simulink model "CryoDetMultiChan_CMB"  (R2016b)
settings: Solver=ode45  StartTime=0.0  StopTime=400e-6  MaxStep=Tclk/4  RelTol=1e-3
values from neighbouring files (symbols this model uses):
  ds_axi = 16    [setupCryoFPGA_CMB.m]
  Fclk = Fadc    (= 307200000)    [setupCryoFPGA_CMB.m]
  lpf = tf(num,den)    [setupCryoFPGA_CMB.m]
  Tclk = 1/Fclk    (= 3.25520833333e-09)    [setupCryoFPGA_CMB.m]
  Ts = 1/Fs    (= 3.25520833333e-09)    [setupADCtoDACloopback.m]    (also in setupCryoFPGA_CMB.m)
undefined symbols (not defined in the file or in its folder): AXI4, i, Lite, xlipgetpartsetting
libraries: xbsIndex_r4 x2215, hdlsllib x6, simulink x3, CryoDetLib x2
(part 2 of 16)

== system CryoDetMultiChan_CMB/DspCore/DAC_fs_LO_Regs ==
  "dfs_LO 0 " : Inport
  dfs_LO 1 : Inport  Port=2
  dfs_LO 2 : Inport  Port=3
  dfs_LO 3 : Inport  Port=4
  dfs_LO 4 : Inport  Port=5
  dfs_LO 5 : Inport  Port=6
  dfs_LO 6 : Inport  Port=7
  dfs_LO 7 : Inport  Port=8
  dfs_LO 8 : Inport  Port=9
  dfs_LO 9 : Inport  Port=10
  dfs_LO 10 : Inport  Port=11
  dfs_LO 11 : Inport  Port=12
  dfs_LO 12 : Inport  Port=13
  dfs_LO 13 : Inport  Port=14
  dfs_LO 14 : Inport  Port=15
  dfs_LO 15 : Inport  Port=16
  BitBasher1 : xbsIndex_r4/BitBasher  bitexpr=a={b[15:0]}  display_expr=on  sr_1=a  arith_type1=Unsigned  bin_pt1=16  sr_2=2  arith_type2=Unsigned  bin_pt2=0  sr_3=3  arith_type3=Unsigned  bin_pt3=0  sr_4=4  arith_type4=Unsigned  bin_pt4=0  dbl_ovrd=off  block_type=bitbasher
  BitBasher{2..11,14,17..20} (15 alike) : xbsIndex_r4/BitBasher  bitexpr=a={b[24:0]}  display_expr=on  sr_1=a  arith_type1=Unsigned  bin_pt1=0  sr_2=2  arith_type2=Unsigned  bin_pt2=0  sr_3=3  arith_type3=Unsigned  bin_pt3=0  sr_4=4  arith_type4=Unsigned  bin_pt4=0  dbl_ovrd=off  block_type=bitbasher
  DSPcore_IO48 : xbsIndex_r4/Gateway In  gui_display_data_type=Fixed-point  arith_type=Unsigned  n_bits=32  bin_pt=0  preci_type=Single  exp_width=8  frac_width=24  rows=1  columns=1  quantization=Truncate  overflow=Wrap  period=Tclk*ds_axi  UseAsADC=off  ADCChannel='1'  interface=AXI4-Lite  automatic_assignment=off  address_offset=hex2dec('B00')  intf_name=''  intf_description=''  default_value=0  timing_constraint=None  locs_specified=off  LOCs={}  io_standard={}  inherit_from_input=off  hdl_port=on  dbl_ovrd=off  block_type=gatewayin
  DSPcore_IO49 : xbsIndex_r4/Gateway In  gui_display_data_type=Fixed-point  arith_type=Unsigned  n_bits=32  bin_pt=0  preci_type=Single  exp_width=8  frac_width=24  rows=1  columns=1  quantization=Truncate  overflow=Wrap  period=Tclk*ds_axi  UseAsADC=off  ADCChannel='1'  interface=AXI4-Lite  automatic_assignment=off  address_offset=hex2dec('B04')  intf_name=''  intf_description=''  default_value=0  timing_constraint=None  locs_specified=off  LOCs={}  io_standard={}  inherit_from_input=off  hdl_port=on  dbl_ovrd=off  block_type=gatewayin
  DSPcore_IO50 : xbsIndex_r4/Gateway In  gui_display_data_type=Fixed-point  arith_type=Unsigned  n_bits=32  bin_pt=0  preci_type=Single  exp_width=8  frac_width=24  rows=1  columns=1  quantization=Truncate  overflow=Wrap  period=Tclk*ds_axi  UseAsADC=off  ADCChannel='1'  interface=AXI4-Lite  automatic_assignment=off  address_offset=hex2dec('B28')  intf_name=''  intf_description=''  default_value=0  timing_constraint=None  locs_specified=off  LOCs={}  io_standard={}  inherit_from_input=off  hdl_port=on  dbl_ovrd=off  block_type=gatewayin
  DSPcore_IO51 : xbsIndex_r4/Gateway In  gui_display_data_type=Fixed-point  arith_type=Unsigned  n_bits=32  bin_pt=0  preci_type=Single  exp_width=8  frac_width=24  rows=1  columns=1  quantization=Truncate  overflow=Wrap  period=Tclk*ds_axi  UseAsADC=off  ADCChannel='1'  interface=AXI4-Lite  automatic_assignment=off  address_offset=hex2dec('B2C')  intf_name=''  intf_description=''  default_value=0  timing_constraint=None  locs_specified=off  LOCs={}  io_standard={}  inherit_from_input=off  hdl_port=on  dbl_ovrd=off  block_type=gatewayin
  DSPcore_IO52 : xbsIndex_r4/Gateway In  gui_display_data_type=Fixed-point  arith_type=Unsigned  n_bits=32  bin_pt=0  preci_type=Single  exp_width=8  frac_width=24  rows=1  columns=1  quantization=Truncate  overflow=Wrap  period=Tclk*ds_axi  UseAsADC=off  ADCChannel='1'  interface=AXI4-Lite  automatic_assignment=off  address_offset=hex2dec('B30')  intf_name=''  intf_description=''  default_value=0  timing_constraint=None  locs_specified=off  LOCs={}  io_standard={}  inherit_from_input=off  hdl_port=on  dbl_ovrd=off  block_type=gatewayin
  DSPcore_IO53 : xbsIndex_r4/Gateway In  gui_display_data_type=Fixed-point  arith_type=Unsigned  n_bits=32  bin_pt=0  preci_type=Single  exp_width=8  frac_width=24  rows=1  columns=1  quantization=Truncate  overflow=Wrap  period=Tclk*ds_axi  UseAsADC=off  ADCChannel='1'  interface=AXI4-Lite  automatic_assignment=off  address_offset=hex2dec('B34')  intf_name=''  intf_description=''  default_value=0  timing_constraint=None  locs_specified=off  LOCs={}  io_standard={}  inherit_from_input=off  hdl_port=on  dbl_ovrd=off  block_type=gatewayin
  DSPcore_IO54 : xbsIndex_r4/Gateway In  gui_display_data_type=Fixed-point  arith_type=Unsigned  n_bits=32  bin_pt=0  preci_type=Single  exp_width=8  frac_width=24  rows=1  columns=1  quantization=Truncate  overflow=Wrap  period=Tclk*ds_axi  UseAsADC=off  ADCChannel='1'  interface=AXI4-Lite  automatic_assignment=off  address_offset=hex2dec('B38')  intf_name=''  intf_description=''  default_value=0  timing_constraint=None  locs_specified=off  LOCs={}  io_standard={}  inherit_from_input=off  hdl_port=on  dbl_ovrd=off  block_type=gatewayin
  DSPcore_IO55 : xbsIndex_r4/Gateway In  gui_display_data_type=Fixed-point  arith_type=Unsigned  n_bits=32  bin_pt=0  preci_type=Single  exp_width=8  frac_width=24  rows=1  columns=1  quantization=Truncate  overflow=Wrap  period=Tclk*ds_axi  UseAsADC=off  ADCChannel='1'  interface=AXI4-Lite  automatic_assignment=off  address_offset=hex2dec('B3C')  intf_name=''  intf_description=''  default_value=0  timing_constraint=None  locs_specified=off  LOCs={}  io_standard={}  inherit_from_input=off  hdl_port=on  dbl_ovrd=off  block_type=gatewayin
  DSPcore_IO56 : xbsIndex_r4/Gateway In  gui_display_data_type=Fixed-point  arith_type=Unsigned  n_bits=32  bin_pt=0  preci_type=Single  exp_width=8  frac_width=24  rows=1  columns=1  quantization=Truncate  overflow=Wrap  period=Tclk*ds_axi  UseAsADC=off  ADCChannel='1'  interface=AXI4-Lite  automatic_assignment=off  address_offset=hex2dec('B08')  intf_name=''  intf_description=''  default_value=0  timing_constraint=None  locs_specified=off  LOCs={}  io_standard={}  inherit_from_input=off  hdl_port=on  dbl_ovrd=off  block_type=gatewayin
  DSPcore_IO57 : xbsIndex_r4/Gateway In  gui_display_data_type=Fixed-point  arith_type=Unsigned  n_bits=32  bin_pt=0  preci_type=Single  exp_width=8  frac_width=24  rows=1  columns=1  quantization=Truncate  overflow=Wrap  period=Tclk*ds_axi  UseAsADC=off  ADCChannel='1'  interface=AXI4-Lite  automatic_assignment=off  address_offset=hex2dec('B0C')  intf_name=''  intf_description=''  default_value=0  timing_constraint=None  locs_specified=off  LOCs={}  io_standard={}  inherit_from_input=off  hdl_port=on  dbl_ovrd=off  block_type=gatewayin
  DSPcore_IO58 : xbsIndex_r4/Gateway In  gui_display_data_type=Fixed-point  arith_type=Unsigned  n_bits=32  bin_pt=0  preci_type=Single  exp_width=8  frac_width=24  rows=1  columns=1  quantization=Truncate  overflow=Wrap  period=Tclk*ds_axi  UseAsADC=off  ADCChannel='1'  interface=AXI4-Lite  automatic_assignment=off  address_offset=hex2dec('B10')  intf_name=''  intf_description=''  default_value=0  timing_constraint=None  locs_specified=off  LOCs={}  io_standard={}  inherit_from_input=off  hdl_port=on  dbl_ovrd=off  block_type=gatewayin
  DSPcore_IO59 : xbsIndex_r4/Gateway In  gui_display_data_type=Fixed-point  arith_type=Unsigned  n_bits=32  bin_pt=0  preci_type=Single  exp_width=8  frac_width=24  rows=1  columns=1  quantization=Truncate  overflow=Wrap  period=Tclk*ds_axi  UseAsADC=off  ADCChannel='1'  interface=AXI4-Lite  automatic_assignment=off  address_offset=hex2dec('B14')  intf_name=''  intf_description=''  default_value=0  timing_constraint=None  locs_specified=off  LOCs={}  io_standard={}  inherit_from_input=off  hdl_port=on  dbl_ovrd=off  block_type=gatewayin
  DSPcore_IO60 : xbsIndex_r4/Gateway In  gui_display_data_type=Fixed-point  arith_type=Unsigned  n_bits=32  bin_pt=0  preci_type=Single  exp_width=8  frac_width=24  rows=1  columns=1  quantization=Truncate  overflow=Wrap  period=Tclk*ds_axi  UseAsADC=off  ADCChannel='1'  interface=AXI4-Lite  automatic_assignment=off  address_offset=hex2dec('B18')  intf_name=''  intf_description=''  default_value=0  timing_constraint=None  locs_specified=off  LOCs={}  io_standard={}  inherit_from_input=off  hdl_port=on  dbl_ovrd=off  block_type=gatewayin
  DSPcore_IO61 : xbsIndex_r4/Gateway In  gui_display_data_type=Fixed-point  arith_type=Unsigned  n_bits=32  bin_pt=0  preci_type=Single  exp_width=8  frac_width=24  rows=1  columns=1  quantization=Truncate  overflow=Wrap  period=Tclk*ds_axi  UseAsADC=off  ADCChannel='1'  interface=AXI4-Lite  automatic_assignment=off  address_offset=hex2dec('B1C')  intf_name=''  intf_description=''  default_value=0  timing_constraint=None  locs_specified=off  LOCs={}  io_standard={}  inherit_from_input=off  hdl_port=on  dbl_ovrd=off  block_type=gatewayin
  DSPcore_IO62 : xbsIndex_r4/Gateway In  gui_display_data_type=Fixed-point  arith_type=Unsigned  n_bits=32  bin_pt=0  preci_type=Single  exp_width=8  frac_width=24  rows=1  columns=1  quantization=Truncate  overflow=Wrap  period=Tclk*ds_axi  UseAsADC=off  ADCChannel='1'  interface=AXI4-Lite  automatic_assignment=off  address_offset=hex2dec('B20')  intf_name=''  intf_description=''  default_value=0  timing_constraint=None  locs_specified=off  LOCs={}  io_standard={}  inherit_from_input=off  hdl_port=on  dbl_ovrd=off  block_type=gatewayin
  DSPcore_IO63 : xbsIndex_r4/Gateway In  gui_display_data_type=Fixed-point  arith_type=Unsigned  n_bits=32  bin_pt=0  preci_type=Single  exp_width=8  frac_width=24  rows=1  columns=1  quantization=Truncate  overflow=Wrap  period=Tclk*ds_axi  UseAsADC=off  ADCChannel='1'  interface=AXI4-Lite  automatic_assignment=off  address_offset=hex2dec('B24')  intf_name=''  intf_description=''  default_value=0  timing_constraint=None  locs_specified=off  LOCs={}  io_standard={}  inherit_from_input=off  hdl_port=on  dbl_ovrd=off  block_type=gatewayin
  F{0..3} (4 alike) : Display
  Gateway Out{,2..4} (4 alike) : xbsIndex_r4/Gateway Out  inherit_from_input=on  hdl_port=off  rows=1  columns=1  UseAsDAC=off  DACChannel='1'  interface=None  automatic_assignment=on  address_offset=hex2dec('00')  intf_name=''  intf_description=''  timing_constraint=None  locs_specified=off  LOCs={}  io_standard={}  block_type=gatewayout
  pipeline_2r : Subsystem
  pipeline_2r1 : Subsystem
  pipeline_2r10 : Subsystem
  pipeline_2r11 : Subsystem
  pipeline_2r12 : Subsystem
  pipeline_2r13 : Subsystem
  pipeline_2r14 : Subsystem
  pipeline_2r15 : Subsystem
  pipeline_2r2 : Subsystem
  pipeline_2r3 : Subsystem
  pipeline_2r4 : Subsystem
  pipeline_2r5 : Subsystem
  pipeline_2r6 : Subsystem
  pipeline_2r7 : Subsystem
  pipeline_2r8 : Subsystem
  pipeline_2r9 : Subsystem
  tag scope: dfs_LO0=global, dfs_LO10=global, dfs_LO11=global, dfs_LO12=global, dfs_LO13=global, dfs_LO14=global, dfs_LO15=global, dfs_LO1=global, dfs_LO2=global, dfs_LO3=global, dfs_LO4=global, dfs_LO5=global, dfs_LO6=global, dfs_LO7=global, dfs_LO8=global, dfs_LO9=global
  wires:
  dfs_LO 14/1 -> DSPcore_IO54/1
  BitBasher5/1 -> [dfs_LO4]
  DSPcore_IO58/1 -> pipeline_2r4/1(In1)
  BitBasher17/1 -> [dfs_LO13]
  dfs_LO 13/1 -> DSPcore_IO53/1
  DSPcore_IO59/1 -> pipeline_2r5/1(In1)
  dfs_LO 15/1 -> DSPcore_IO55/1
  BitBasher11/1 -> [dfs_LO10]
  dfs_LO 7/1 -> DSPcore_IO61/1
  dfs_LO 11/1 -> DSPcore_IO51/1
  dfs_LO 9/1 -> DSPcore_IO63/1
  Gateway Out4/1 -> F3/1
  BitBasher4/1 -> [dfs_LO3], Gateway Out4/1
  dfs_LO 5/1 -> DSPcore_IO59/1
  DSPcore_IO55/1 -> pipeline_2r15/1(In1)
  DSPcore_IO53/1 -> pipeline_2r13/1(In1)
  DSPcore_IO63/1 -> pipeline_2r9/1(In1)
  BitBasher6/1 -> [dfs_LO5]
  dfs_LO 8/1 -> DSPcore_IO62/1
  DSPcore_IO52/1 -> pipeline_2r12/1(In1)
  BitBasher20/1 -> [dfs_LO12]
  DSPcore_IO57/1 -> pipeline_2r3/1(In1)
  dfs_LO 4/1 -> DSPcore_IO58/1
  Gateway Out2/1 -> F1/1
  BitBasher2/1 -> [dfs_LO1], Gateway Out2/1
  DSPcore_IO62/1 -> pipeline_2r8/1(In1)
  BitBasher14/1 -> [dfs_LO11]
  BitBasher19/1 -> [dfs_LO15]
  dfs_LO 10/1 -> DSPcore_IO50/1
  BitBasher10/1 -> [dfs_LO9]
  DSPcore_IO51/1 -> pipeline_2r11/1(In1)
  DSPcore_IO56/1 -> pipeline_2r2/1(In1)
  dfs_LO 2/1 -> DSPcore_IO56/1
  Gateway Out3/1 -> F2/1
  BitBasher3/1 -> [dfs_LO2], Gateway Out3/1
  DSPcore_IO54/1 -> pipeline_2r14/1(In1)
  DSPcore_IO49/1 -> pipeline_2r1/1(In1)
  dfs_LO 1/1 -> DSPcore_IO49/1
  BitBasher9/1 -> [dfs_LO8]
  DSPcore_IO61/1 -> pipeline_2r7/1(In1)
  BitBasher18/1 -> [dfs_LO14]
  DSPcore_IO50/1 -> pipeline_2r10/1(In1)
  dfs_LO 6/1 -> DSPcore_IO60/1
  dfs_LO 3/1 -> DSPcore_IO57/1
  "dfs_LO 0 "/1 -> DSPcore_IO48/1
  Gateway Out/1 -> F0/1
  BitBasher1/1 -> [dfs_LO0], Gateway Out/1
  DSPcore_IO48/1 -> pipeline_2r/1(In1)
  BitBasher7/1 -> [dfs_LO6]
  BitBasher8/1 -> [dfs_LO7]
  dfs_LO 12/1 -> DSPcore_IO52/1
  DSPcore_IO60/1 -> pipeline_2r6/1(In1)
  pipeline_2r/1(Out1) -> BitBasher1/1
  pipeline_2r1/1(Out1) -> BitBasher2/1
  pipeline_2r2/1(Out1) -> BitBasher3/1
  pipeline_2r3/1(Out1) -> BitBasher4/1
  pipeline_2r5/1(Out1) -> BitBasher6/1
  pipeline_2r4/1(Out1) -> BitBasher5/1
  pipeline_2r6/1(Out1) -> BitBasher7/1
  pipeline_2r7/1(Out1) -> BitBasher8/1
  pipeline_2r9/1(Out1) -> BitBasher10/1
  pipeline_2r10/1(Out1) -> BitBasher11/1
  pipeline_2r8/1(Out1) -> BitBasher9/1
  pipeline_2r11/1(Out1) -> BitBasher14/1
  pipeline_2r13/1(Out1) -> BitBasher17/1
  pipeline_2r14/1(Out1) -> BitBasher18/1
  pipeline_2r12/1(Out1) -> BitBasher20/1
  pipeline_2r15/1(Out1) -> BitBasher19/1

== system CryoDetMultiChan_CMB/DspCore/FTA_Ch0 ==
  note: Band B is not used for now..
  note: reference
  ADCin_A : Inport
  ADCin_B : Inport  Port=2
  ADC_IQ_Swap : Subsystem
  DAC_Output_Fmt : Subsystem
  Goto Tag Visibility : GotoTagVisibility  GotoTag=freqBus
  Goto Tag Visibility1 : GotoTagVisibility  GotoTag=dphiBus
  Goto Tag Visibility2 : GotoTagVisibility  GotoTag=dFbus
  RF switch : Subsystem
  Ref Delay : Subsystem
  SixteenLineUDC 0 : Subsystem
  Terminator : Terminator
  Terminator1 : Terminator
  dF : Subsystem
  dphi : Subsystem
  loopFilter : Subsystem
  shiftFreq : Subsystem
  twelveLineUDC 1 : Subsystem
  DAC_I_out : Outport
  DAC_Q_out : Outport  Port=2
  wires:
  twelveLineUDC 1/1(Out1) -> Terminator/1
  SixteenLineUDC 0/1(toDAC) -> RF switch/1(In1)
  SixteenLineUDC 0/2(demodulated) -> dF/1(In1)
  dF/1(Out1) -> loopFilter/1(In1)
  loopFilter/1(Out1) -> dphi/1(In1)
  ADCin_B/1 -> Terminator1/1
  [Band1_IQ_In_Swap] -> ADC_IQ_Swap/1(Swap_en)
  ADCin_A/1 -> ADC_IQ_Swap/2(ADC_in)
  ADC_IQ_Swap/1(ADC_I_out) -> SixteenLineUDC 0/1(ADC_I_in)
  ADC_IQ_Swap/2(ADC_Q_out) -> SixteenLineUDC 0/2(ADC_Q_in)
  shiftFreq/1(Out1) -> DAC_Output_Fmt/1(In1)
  DAC_Output_Fmt/1(Out_Q) -> DAC_Q_out/1
  DAC_Output_Fmt/2(Out_I) -> DAC_I_out/1
  Ref Delay/1(Out_Q) -> SixteenLineUDC 0/4(REF_Q_in1)
  Ref Delay/2(Out_I) -> SixteenLineUDC 0/3(REF_I_in1)
  RF switch/1(to_DAC) -> shiftFreq/1(In1)
  RF switch/2(to_REF) -> Ref Delay/1(In1)

== system CryoDetMultiChan_CMB/DspCore/FTA_Ch1 ==
  note: FTA Ch1
      | Only a pass thu for now...
      |
      | Note that this type of 1:1 connection ONLY works
      | when the ADC is in Single-Band Complex mode b/c
      | of how the adc data is mapped.
      | This is here for testing only.
  ADCin_A : Inport
  ADCin_B : Inport  Port=2
  DAC_I_out : Outport
  DAC_Q_out : Outport  Port=2
  wires:
  ADCin_A/1 -> DAC_I_out/1
  ADCin_B/1 -> DAC_Q_out/1

== system CryoDetMultiChan_CMB/DspCore/Initial_Freq_Regs ==
  "Fi 0 " : Inport
  Fi 1 : Inport  Port=2
  Fi 2 : Inport  Port=3
  Fi 3 : Inport  Port=4
  Fi 4 : Inport  Port=5
  Fi 5 : Inport  Port=6
  Fi 6 : Inport  Port=7
  Fi 7 : Inport  Port=8
  Fi 8 : Inport  Port=9
  Fi 9 : Inport  Port=10
  Fi 10 : Inport  Port=11
  Fi 11 : Inport  Port=12
  Fi 12 : Inport  Port=13
  Fi 13 : Inport  Port=14
  Fi 14 : Inport  Port=15
  Fi 15 : Inport  Port=16
  BitBasher{1..11,14,17..20} (16 alike) : xbsIndex_r4/BitBasher  bitexpr=a={b[24:0]}  display_expr=on  sr_1=a  arith_type1=Unsigned  bin_pt1=0  sr_2=2  arith_type2=Unsigned  bin_pt2=0  sr_3=3  arith_type3=Unsigned  bin_pt3=0  sr_4=4  arith_type4=Unsigned  bin_pt4=0  dbl_ovrd=off  block_type=bitbasher
  DSPcore_IO : xbsIndex_r4/Gateway In  gui_display_data_type=Fixed-point  arith_type=Unsigned  n_bits=32  bin_pt=0  preci_type=Single  exp_width=8  frac_width=24  rows=1  columns=1  quantization=Truncate  overflow=Wrap  period=Tclk*ds_axi  UseAsADC=off  ADCChannel='1'  interface=AXI4-Lite  automatic_assignment=off  address_offset=hex2dec('900')  intf_name=''  intf_description=''  default_value=0  timing_constraint=None  locs_specified=off  LOCs={}  io_standard={}  inherit_from_input=off  hdl_port=on  dbl_ovrd=off  block_type=gatewayin
  DSPcore_IO1 : xbsIndex_r4/Gateway In  gui_display_data_type=Fixed-point  arith_type=Unsigned  n_bits=32  bin_pt=0  preci_type=Single  exp_width=8  frac_width=24  rows=1  columns=1  quantization=Truncate  overflow=Wrap  period=Tclk*ds_axi  UseAsADC=off  ADCChannel='1'  interface=AXI4-Lite  automatic_assignment=off  address_offset=hex2dec('904')  intf_name=''  intf_description=''  default_value=0  timing_constraint=None  locs_specified=off  LOCs={}  io_standard={}  inherit_from_input=off  hdl_port=on  dbl_ovrd=off  block_type=gatewayin
  DSPcore_IO10 : xbsIndex_r4/Gateway In  gui_display_data_type=Fixed-point  arith_type=Unsigned  n_bits=32  bin_pt=0  preci_type=Single  exp_width=8  frac_width=24  rows=1  columns=1  quantization=Truncate  overflow=Wrap  period=Tclk*ds_axi  UseAsADC=off  ADCChannel='1'  interface=AXI4-Lite  automatic_assignment=off  address_offset=hex2dec('928')  intf_name=''  intf_description=''  default_value=0  timing_constraint=None  locs_specified=off  LOCs={}  io_standard={}  inherit_from_input=off  hdl_port=on  dbl_ovrd=off  block_type=gatewayin
  DSPcore_IO11 : xbsIndex_r4/Gateway In  gui_display_data_type=Fixed-point  arith_type=Unsigned  n_bits=32  bin_pt=0  preci_type=Single  exp_width=8  frac_width=24  rows=1  columns=1  quantization=Truncate  overflow=Wrap  period=Tclk*ds_axi  UseAsADC=off  ADCChannel='1'  interface=AXI4-Lite  automatic_assignment=off  address_offset=hex2dec('92C')  intf_name=''  intf_description=''  default_value=0  timing_constraint=None  locs_specified=off  LOCs={}  io_standard={}  inherit_from_input=off  hdl_port=on  dbl_ovrd=off  block_type=gatewayin
  DSPcore_IO12 : xbsIndex_r4/Gateway In  gui_display_data_type=Fixed-point  arith_type=Unsigned  n_bits=32  bin_pt=0  preci_type=Single  exp_width=8  frac_width=24  rows=1  columns=1  quantization=Truncate  overflow=Wrap  period=Tclk*ds_axi  UseAsADC=off  ADCChannel='1'  interface=AXI4-Lite  automatic_assignment=off  address_offset=hex2dec('930')  intf_name=''  intf_description=''  default_value=0  timing_constraint=None  locs_specified=off  LOCs={}  io_standard={}  inherit_from_input=off  hdl_port=on  dbl_ovrd=off  block_type=gatewayin
  DSPcore_IO13 : xbsIndex_r4/Gateway In  gui_display_data_type=Fixed-point  arith_type=Unsigned  n_bits=32  bin_pt=0  preci_type=Single  exp_width=8  frac_width=24  rows=1  columns=1  quantization=Truncate  overflow=Wrap  period=Tclk*ds_axi  UseAsADC=off  ADCChannel='1'  interface=AXI4-Lite  automatic_assignment=off  address_offset=hex2dec('934')  intf_name=''  intf_description=''  default_value=0  timing_constraint=None  locs_specified=off  LOCs={}  io_standard={}  inherit_from_input=off  hdl_port=on  dbl_ovrd=off  block_type=gatewayin
  DSPcore_IO14 : xbsIndex_r4/Gateway In  gui_display_data_type=Fixed-point  arith_type=Unsigned  n_bits=32  bin_pt=0  preci_type=Single  exp_width=8  frac_width=24  rows=1  columns=1  quantization=Truncate  overflow=Wrap  period=Tclk*ds_axi  UseAsADC=off  ADCChannel='1'  interface=AXI4-Lite  automatic_assignment=off  address_offset=hex2dec('938')  intf_name=''  intf_description=''  default_value=0  timing_constraint=None  locs_specified=off  LOCs={}  io_standard={}  inherit_from_input=off  hdl_port=on  dbl_ovrd=off  block_type=gatewayin
  DSPcore_IO15 : xbsIndex_r4/Gateway In  gui_display_data_type=Fixed-point  arith_type=Unsigned  n_bits=32  bin_pt=0  preci_type=Single  exp_width=8  frac_width=24  rows=1  columns=1  quantization=Truncate  overflow=Wrap  period=Tclk*ds_axi  UseAsADC=off  ADCChannel='1'  interface=AXI4-Lite  automatic_assignment=off  address_offset=hex2dec('93C')  intf_name=''  intf_description=''  default_value=0  timing_constraint=None  locs_specified=off  LOCs={}  io_standard={}  inherit_from_input=off  hdl_port=on  dbl_ovrd=off  block_type=gatewayin
  DSPcore_IO2 : xbsIndex_r4/Gateway In  gui_display_data_type=Fixed-point  arith_type=Unsigned  n_bits=32  bin_pt=0  preci_type=Single  exp_width=8  frac_width=24  rows=1  columns=1  quantization=Truncate  overflow=Wrap  period=Tclk*ds_axi  UseAsADC=off  ADCChannel='1'  interface=AXI4-Lite  automatic_assignment=off  address_offset=hex2dec('908')  intf_name=''  intf_description=''  default_value=0  timing_constraint=None  locs_specified=off  LOCs={}  io_standard={}  inherit_from_input=off  hdl_port=on  dbl_ovrd=off  block_type=gatewayin
  DSPcore_IO3 : xbsIndex_r4/Gateway In  gui_display_data_type=Fixed-point  arith_type=Unsigned  n_bits=32  bin_pt=0  preci_type=Single  exp_width=8  frac_width=24  rows=1  columns=1  quantization=Truncate  overflow=Wrap  period=Tclk*ds_axi  UseAsADC=off  ADCChannel='1'  interface=AXI4-Lite  automatic_assignment=off  address_offset=hex2dec('90C')  intf_name=''  intf_description=''  default_value=0  timing_constraint=None  locs_specified=off  LOCs={}  io_standard={}  inherit_from_input=off  hdl_port=on  dbl_ovrd=off  block_type=gatewayin
  DSPcore_IO4 : xbsIndex_r4/Gateway In  gui_display_data_type=Fixed-point  arith_type=Unsigned  n_bits=32  bin_pt=0  preci_type=Single  exp_width=8  frac_width=24  rows=1  columns=1  quantization=Truncate  overflow=Wrap  period=Tclk*ds_axi  UseAsADC=off  ADCChannel='1'  interface=AXI4-Lite  automatic_assignment=off  address_offset=hex2dec('910')  intf_name=''  intf_description=''  default_value=0  timing_constraint=None  locs_specified=off  LOCs={}  io_standard={}  inherit_from_input=off  hdl_port=on  dbl_ovrd=off  block_type=gatewayin
  DSPcore_IO5 : xbsIndex_r4/Gateway In  gui_display_data_type=Fixed-point  arith_type=Unsigned  n_bits=32  bin_pt=0  preci_type=Single  exp_width=8  frac_width=24  rows=1  columns=1  quantization=Truncate  overflow=Wrap  period=Tclk*ds_axi  UseAsADC=off  ADCChannel='1'  interface=AXI4-Lite  automatic_assignment=off  address_offset=hex2dec('914')  intf_name=''  intf_description=''  default_value=0  timing_constraint=None  locs_specified=off  LOCs={}  io_standard={}  inherit_from_input=off  hdl_port=on  dbl_ovrd=off  block_type=gatewayin
  DSPcore_IO6 : xbsIndex_r4/Gateway In  gui_display_data_type=Fixed-point  arith_type=Unsigned  n_bits=32  bin_pt=0  preci_type=Single  exp_width=8  frac_width=24  rows=1  columns=1  quantization=Truncate  overflow=Wrap  period=Tclk*ds_axi  UseAsADC=off  ADCChannel='1'  interface=AXI4-Lite  automatic_assignment=off  address_offset=hex2dec('918')  intf_name=''  intf_description=''  default_value=0  timing_constraint=None  locs_specified=off  LOCs={}  io_standard={}  inherit_from_input=off  hdl_port=on  dbl_ovrd=off  block_type=gatewayin
  DSPcore_IO7 : xbsIndex_r4/Gateway In  gui_display_data_type=Fixed-point  arith_type=Unsigned  n_bits=32  bin_pt=0  preci_type=Single  exp_width=8  frac_width=24  rows=1  columns=1  quantization=Truncate  overflow=Wrap  period=Tclk*ds_axi  UseAsADC=off  ADCChannel='1'  interface=AXI4-Lite  automatic_assignment=off  address_offset=hex2dec('91C')  intf_name=''  intf_description=''  default_value=0  timing_constraint=None  locs_specified=off  LOCs={}  io_standard={}  inherit_from_input=off  hdl_port=on  dbl_ovrd=off  block_type=gatewayin
  DSPcore_IO8 : xbsIndex_r4/Gateway In  gui_display_data_type=Fixed-point  arith_type=Unsigned  n_bits=32  bin_pt=0  preci_type=Single  exp_width=8  frac_width=24  rows=1  columns=1  quantization=Truncate  overflow=Wrap  period=Tclk*ds_axi  UseAsADC=off  ADCChannel='1'  interface=AXI4-Lite  automatic_assignment=off  address_offset=hex2dec('920')  intf_name=''  intf_description=''  default_value=0  timing_constraint=None  locs_specified=off  LOCs={}  io_standard={}  inherit_from_input=off  hdl_port=on  dbl_ovrd=off  block_type=gatewayin
  DSPcore_IO9 : xbsIndex_r4/Gateway In  gui_display_data_type=Fixed-point  arith_type=Unsigned  n_bits=32  bin_pt=0  preci_type=Single  exp_width=8  frac_width=24  rows=1  columns=1  quantization=Truncate  overflow=Wrap  period=Tclk*ds_axi  UseAsADC=off  ADCChannel='1'  interface=AXI4-Lite  automatic_assignment=off  address_offset=hex2dec('924')  intf_name=''  intf_description=''  default_value=0  timing_constraint=None  locs_specified=off  LOCs={}  io_standard={}  inherit_from_input=off  hdl_port=on  dbl_ovrd=off  block_type=gatewayin
  F{0..3} (4 alike) : Display
  Gateway Out{,2..4} (4 alike) : xbsIndex_r4/Gateway Out  inherit_from_input=on  hdl_port=off  rows=1  columns=1  UseAsDAC=off  DACChannel='1'  interface=None  automatic_assignment=on  address_offset=hex2dec('00')  intf_name=''  intf_description=''  timing_constraint=None  locs_specified=off  LOCs={}  io_standard={}  block_type=gatewayout
  pipeline_2r : Subsystem
  pipeline_2r1 : Subsystem
  pipeline_2r10 : Subsystem
  pipeline_2r11 : Subsystem
  pipeline_2r12 : Subsystem
  pipeline_2r13 : Subsystem
  pipeline_2r14 : Subsystem
  pipeline_2r15 : Subsystem
  pipeline_2r2 : Subsystem
  pipeline_2r3 : Subsystem
  pipeline_2r4 : Subsystem
  pipeline_2r5 : Subsystem
  pipeline_2r6 : Subsystem
  pipeline_2r7 : Subsystem
  pipeline_2r8 : Subsystem
  pipeline_2r9 : Subsystem
  tag scope: F0=global, F10=global, F11=global, F12=global, F13=global, F14=global, F15=global, F1=global, F2=global, F3=global, F4=global, F5=global, F6=global, F7=global, F8=global, F9=global
  wires:
  Fi 14/1 -> DSPcore_IO14/1
  BitBasher5/1 -> [F4]
  DSPcore_IO4/1 -> pipeline_2r4/1(In1)
  BitBasher17/1 -> [F13]
  Fi 13/1 -> DSPcore_IO13/1
  DSPcore_IO5/1 -> pipeline_2r5/1(In1)
  Fi 15/1 -> DSPcore_IO15/1
  BitBasher11/1 -> [F10]
  Fi 7/1 -> DSPcore_IO7/1
  Fi 11/1 -> DSPcore_IO11/1
  Fi 9/1 -> DSPcore_IO9/1
  Gateway Out4/1 -> F3/1
  BitBasher4/1 -> Gateway Out4/1, [F3]
  Fi 5/1 -> DSPcore_IO5/1
  DSPcore_IO15/1 -> pipeline_2r15/1(In1)
  DSPcore_IO13/1 -> pipeline_2r13/1(In1)
  DSPcore_IO9/1 -> pipeline_2r9/1(In1)
  BitBasher6/1 -> [F5]
  Fi 8/1 -> DSPcore_IO8/1
  DSPcore_IO12/1 -> pipeline_2r12/1(In1)
  BitBasher20/1 -> [F12]
  DSPcore_IO3/1 -> pipeline_2r3/1(In1)
  Fi 4/1 -> DSPcore_IO4/1
  Gateway Out2/1 -> F1/1
  BitBasher2/1 -> [F1], Gateway Out2/1
  DSPcore_IO8/1 -> pipeline_2r8/1(In1)
  BitBasher14/1 -> [F11]
  BitBasher19/1 -> [F15]
  Fi 10/1 -> DSPcore_IO10/1
  BitBasher10/1 -> [F9]
  DSPcore_IO11/1 -> pipeline_2r11/1(In1)
  DSPcore_IO2/1 -> pipeline_2r2/1(In1)
  Fi 2/1 -> DSPcore_IO2/1
  Gateway Out3/1 -> F2/1
  BitBasher3/1 -> [F2], Gateway Out3/1
  DSPcore_IO14/1 -> pipeline_2r14/1(In1)
  DSPcore_IO1/1 -> pipeline_2r1/1(In1)
  Fi 1/1 -> DSPcore_IO1/1
  BitBasher9/1 -> [F8]
  DSPcore_IO7/1 -> pipeline_2r7/1(In1)
  BitBasher18/1 -> [F14]
  DSPcore_IO10/1 -> pipeline_2r10/1(In1)
  Fi 6/1 -> DSPcore_IO6/1
  Fi 3/1 -> DSPcore_IO3/1
  "Fi 0 "/1 -> DSPcore_IO/1
  Gateway Out/1 -> F0/1
  BitBasher1/1 -> [F0], Gateway Out/1
  DSPcore_IO/1 -> pipeline_2r/1(In1)
  BitBasher7/1 -> [F6]
  BitBasher8/1 -> [F7]
  Fi 12/1 -> DSPcore_IO12/1
  DSPcore_IO6/1 -> pipeline_2r6/1(In1)
  pipeline_2r/1(Out1) -> BitBasher1/1
  pipeline_2r1/1(Out1) -> BitBasher2/1
  pipeline_2r2/1(Out1) -> BitBasher3/1
  pipeline_2r3/1(Out1) -> BitBasher4/1
  pipeline_2r5/1(Out1) -> BitBasher6/1
  pipeline_2r7/1(Out1) -> BitBasher8/1
  pipeline_2r6/1(Out1) -> BitBasher7/1
  pipeline_2r4/1(Out1) -> BitBasher5/1
  pipeline_2r11/1(Out1) -> BitBasher14/1
  pipeline_2r8/1(Out1) -> BitBasher9/1
  pipeline_2r10/1(Out1) -> BitBasher11/1
  pipeline_2r9/1(Out1) -> BitBasher10/1
  pipeline_2r15/1(Out1) -> BitBasher19/1
  pipeline_2r12/1(Out1) -> BitBasher20/1
  pipeline_2r14/1(Out1) -> BitBasher18/1
  pipeline_2r13/1(Out1) -> BitBasher17/1

== system CryoDetMultiChan_CMB/DspCore/RTM_IO ==
  In1 : Inport
  Constant : xbsIndex_r4/Constant  const=0  gui_display_data_type=Fixed-point  arith_type=Unsigned  n_bits=16  bin_pt=0  preci_type=Single  exp_width=8  frac_width=24  explicit_period=off  period=1  equ=P=C  opselect=C  inp2=PCIN>>17  opr=+  inp1=P  carry=CIN  dbl_ovrd=off  block_type=constant
  rtmDin : xbsIndex_r4/Gateway In  gui_display_data_type=Fixed-point  arith_type=Unsigned  n_bits=16  bin_pt=0  preci_type=Single  exp_width=8  frac_width=24  rows=1  columns=1  quantization="Round  (unbiased: +/- Inf)"  overflow=Saturate  period=1  UseAsADC=off  ADCChannel='1'  interface=None  automatic_assignment=on  address_offset=hex2dec('00')  intf_name=''  intf_description=''  default_value=0  timing_constraint=None  locs_specified=off  LOCs={}  io_standard={}  inherit_from_input=off  hdl_port=on  dbl_ovrd=off  block_type=gatewayin
  rtmDout : xbsIndex_r4/Gateway Out  inherit_from_input=off  hdl_port=on  rows=1  columns=1  UseAsDAC=off  DACChannel='1'  interface=None  automatic_assignment=on  address_offset=hex2dec('00')  intf_name=''  intf_description=''  timing_constraint=None  locs_specified=off  LOCs={}  io_standard={}  block_type=gatewayout
  Out1 : Outport
  Out2 : Outport  Port=2
  wires:
  Constant/1 -> rtmDout/1
  rtmDout/1 -> Out2/1
  rtmDin/1 -> Out1/1
  In1/1 -> rtmDin/1
